simulink model "sim_2023_A2_inv_pend_OPT"  (R2022b)
settings: Solver=ode45  StartTime=0.0  StopTime=Tf  RelTol=1e-3
StartFcn:
  | sim_inv_pend
values from neighbouring files (symbols this model uses):
  A = sys_dt.A    [main_inv_pend.m]
  AN = [INm ... (first row only)    [gen_mpc_matrices.m]
  B = sys_dt.B    [main_inv_pend.m]
  C = sys_dt.C    [main_inv_pend.m]
  CL = 1    [main_inv_pend.m]
  controller = 1    [main_inv_pend.m]
  F = Phi'*QN*Lambda    [gen_mpc_matrices.m]
  Kf = Kf_t'    [main_inv_pend.m]
  Lambda = zeros(N*n,n)    [gen_mpc_matrices.m]
  N = 1    [gen_mpc_matrices.m]    (also in main_inv_pend.m = 16)
  noise = 1    [main_inv_pend.m]
  obs = 1    [main_inv_pend.m]
  saturate = 0    [main_inv_pend.m]
  th_o = 0    [main_inv_pend.m]
  Ts = 1/20    (= 0.05)    [main_inv_pend.m]
  Umax = [Umax;umax]    [gen_mpc_matrices.m]
  Umin = [Umin;umin]    [gen_mpc_matrices.m]
  W = 1*sqrt(M/5)    [animated_inv_pend_uw_clkw.m]    (also in gen_mpc_matrices.m = (W+W')/2)
  w_o = 0    [main_inv_pend.m]
  x_o = -1    [main_inv_pend.m]
  Xmax = [Xmax;xmax]    [gen_mpc_matrices.m]
  Xmin = [Xmin;xmin]    [gen_mpc_matrices.m]
  xo_hat = [0 0 0 0]'    [main_inv_pend.m]
  xsp_o = 0    [main_inv_pend.m]
undefined symbols (not defined in the file or in its folder): b, g, K, l, Mc, mp
settings Model: Creator=ricardoaguilera  LastModifiedBy=lucien
settings SolverCC: AlgebraicLoopSolver=TrustRegion
settings DataIOCC: ReturnWorkspaceOutputs=off
settings OptimizationCC: LifeSpan=inf
settings DebuggingCC: AlgebraicLoopMsg=none  UnconnectedInputMsg=warning  UnconnectedOutputMsg=warning  UnconnectedLineMsg=warning  SFMachineParentedDataDiag=warning  ArithmeticOperatorsInVariantConditions=warning
settings ModelReferenceCC: EnableRefExpFcnMdlSchedulingChecks=on
settings SFSimCC: CustomCodeUndefinedFunction=UseInterfaceOnly
settings RTWCC: DLArmComputeVersion=19.05
settings CodeAppCC: StateflowObjectComments=on

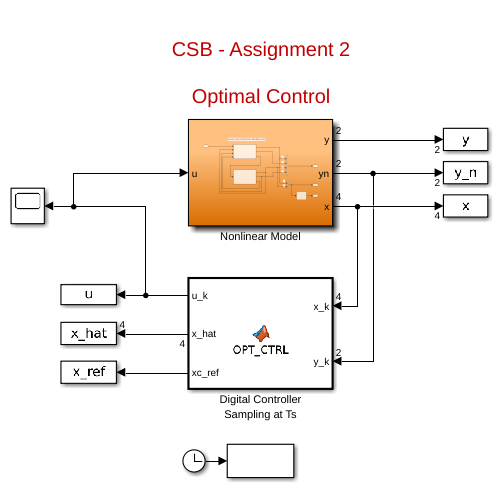
[thumbnail: Simulink's stored preview of the top-level diagram]
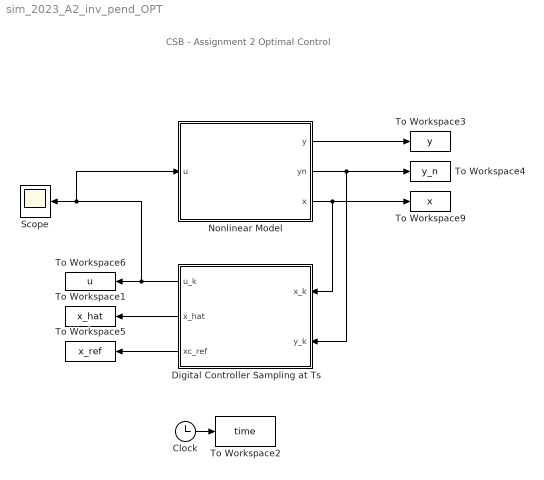
== system sim_2023_A2_inv_pend_OPT ==
  note: CSB - Assignment 2
      |
      | Optimal Control
  Clock : Clock
  Digital Controller Sampling at Ts : MATLAB Function  TreatAsAtomicUnit=on  SystemSampleTime=Ts
  Nonlinear Model : Subsystem
  Scope : Scope
  To Workspace1 : ToWorkspace  VariableName=x_hat  SampleTime=Ts/100
  To Workspace2 : ToWorkspace  VariableName=time  SampleTime=Ts/100
  To Workspace3 : ToWorkspace  VariableName=y  SampleTime=Ts/100
  To Workspace4 : ToWorkspace  VariableName=y_n  SampleTime=Ts/100
  To Workspace5 : ToWorkspace  VariableName=x_ref  SampleTime=Ts/100
  To Workspace6 : ToWorkspace  VariableName=u  SampleTime=Ts/100
  To Workspace9 : ToWorkspace  VariableName=x  SampleTime=Ts/100
  wires:
  Clock/1 -> To Workspace2/1
  Digital Controller Sampling at Ts/2(x_hat) -> To Workspace1/1
  Nonlinear Model/2(yn) -> Digital Controller Sampling at Ts/2(y_k), To Workspace4/1
  Nonlinear Model/3(x) -> Digital Controller Sampling at Ts/1(x_k), To Workspace9/1
  Nonlinear Model/1(y) -> To Workspace3/1
  Digital Controller Sampling at Ts/3(xc_ref) -> To Workspace5/1
  Digital Controller Sampling at Ts/1(u_k) -> To Workspace6/1, Nonlinear Model/1(u), Scope/1

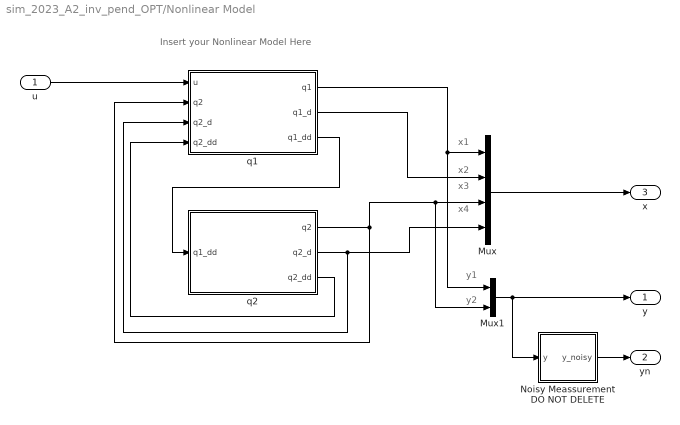
== system sim_2023_A2_inv_pend_OPT/Nonlinear Model ==
  note: x1
  note: Insert your Nonlinear Model Here
  note: x2
  note: x3
  note: x4
  note: y1
  note: y2
  u : Inport
  Mux : Mux
  Mux1 : Mux  Inputs=2
  Noisy Meassurement DO NOT DELETE : Subsystem
  q1 : Subsystem
  q2 : Subsystem
  y : Outport  VectorParamsAs1DForOutWhenUnconnected=off
  yn : Outport  Port=2  VectorParamsAs1DForOutWhenUnconnected=off
  x : Outport  Port=3  VectorParamsAs1DForOutWhenUnconnected=off
  wires:
  q2/3(q2_dd) -> q1/4(q2_dd)
  q2/2(q2_d) -> q1/3(q2_d), Mux/4
  q2/1(q2) -> q1/2(q2), Mux1/2, Mux/3
  q1/2(q1_d) -> Mux/2
  q1/1(q1) -> Mux1/1, Mux/1
  Mux/1 -> x/1
  Mux1/1 -> Noisy Meassurement DO NOT DELETE/1(y), y/1
  u/1 -> q1/1(u)
  Noisy Meassurement DO NOT DELETE/1(y_noisy) -> yn/1
  q1/3(q1_dd) -> q2/1(q1_dd)

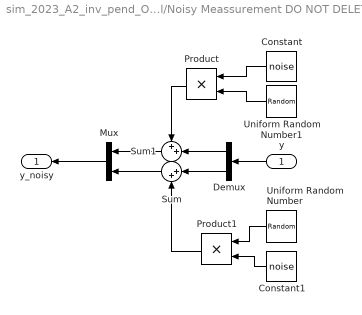
== system sim_2023_A2_inv_pend_OPT/Nonlinear Model/Noisy Meassurement DO NOT DELETE ==
  y : Inport
  Constant : Constant  Value=noise
  Constant1 : Constant  Value=noise
  Demux : Demux  Outputs=2
  Mux : Mux  Inputs=2
  Product : Product
  Product1 : Product
  Sum : Sum  Inputs=|++
  Sum1 : Sum  Inputs=++|
  Uniform Random Number : UniformRandomNumber  Minimum=-0.002  Maximum=0.002  SampleTime=0.5*Ts
  Uniform Random Number1 : UniformRandomNumber  Minimum=-0.3  Maximum=0.3  SampleTime=0.5*Ts
  y_noisy : Outport  VectorParamsAs1DForOutWhenUnconnected=off
  wires:
  Mux/1 -> y_noisy/1
  y/1 -> Demux/1
  Demux/2 -> Sum/1
  Sum/1 -> Mux/2
  Sum1/1 -> Mux/1
  Demux/1 -> Sum1/2
  Constant/1 -> Product/1
  Uniform Random Number1/1 -> Product/2
  Product/1 -> Sum1/1
  Product1/1 -> Sum/2
  Uniform Random Number/1 -> Product1/1
  Constant1/1 -> Product1/2

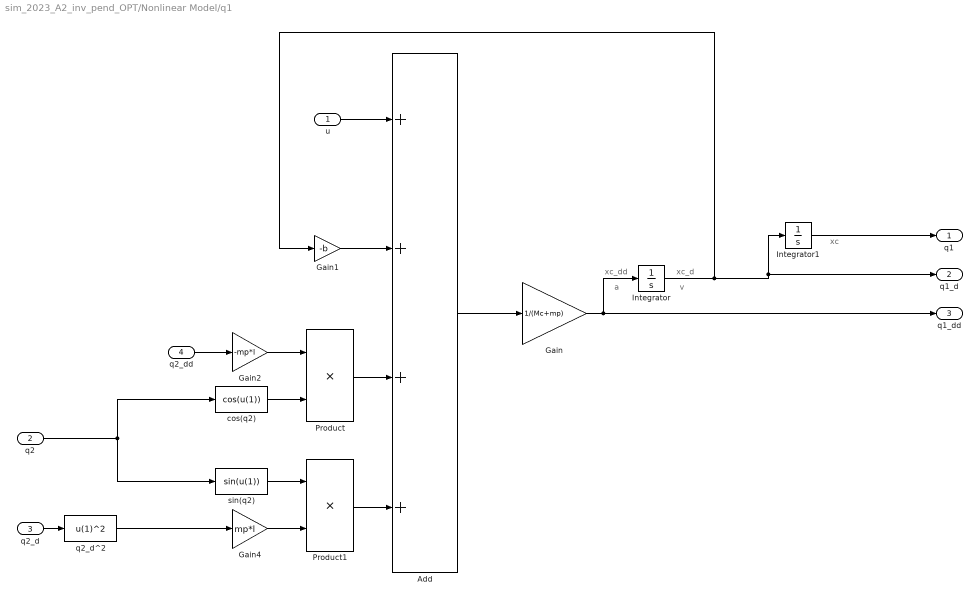
== system sim_2023_A2_inv_pend_OPT/Nonlinear Model/q1 ==
  note: a
  note: xc_dd
  note: v
  note: xc_d
  note: xc
  u : Inport
  q2 : Inport  Port=2
  q2_d : Inport  Port=3
  q2_dd : Inport  Port=4
  Add : Sum  Inputs=++++
  Gain : Gain  Gain=1/(Mc+mp)
  Gain1 : Gain  Gain=-b
  Gain2 : Gain  Gain=-mp*l
  Gain4 : Gain  Gain=mp*l
  Integrator : Integrator  InitialCondition=xsp_o
  Integrator1 : Integrator  InitialCondition=x_o
  Product : Product
  Product1 : Product
  cos(q2) : Fcn  Expr=cos(u(1))
  q2_d^2 : Fcn  Expr=u(1)^2
  sin(q2) : Fcn  Expr=sin(u(1))
  q1 : Outport  VectorParamsAs1DForOutWhenUnconnected=off
  q1_d : Outport  Port=2  VectorParamsAs1DForOutWhenUnconnected=off
  q1_dd : Outport  Port=3  VectorParamsAs1DForOutWhenUnconnected=off
  wires:
  Gain/1 -> Integrator/1, q1_dd/1
  Integrator1/1 -> q1/1
  Integrator/1 -> Gain1/1, q1_d/1, Integrator1/1
  Add/1 -> Gain/1
  u/1 -> Add/1
  Gain1/1 -> Add/2
  Product/1 -> Add/3
  Gain2/1 -> Product/1
  cos(q2)/1 -> Product/2
  Product1/1 -> Add/4
  sin(q2)/1 -> Product1/1
  Gain4/1 -> Product1/2
  q2_d/1 -> q2_d^2/1
  q2_d^2/1 -> Gain4/1
  q2/1 -> sin(q2)/1, cos(q2)/1
  q2_dd/1 -> Gain2/1

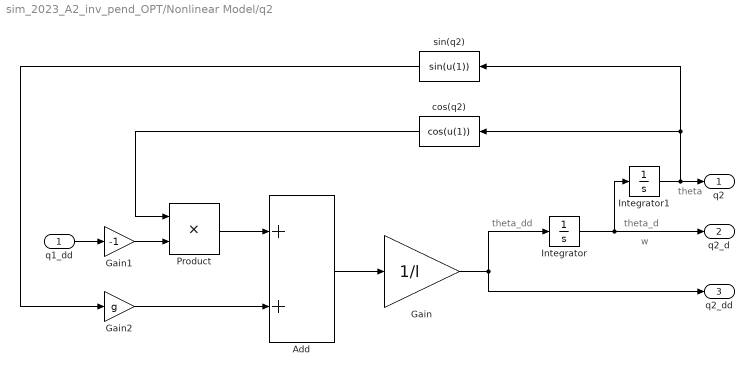
== system sim_2023_A2_inv_pend_OPT/Nonlinear Model/q2 ==
  note: theta_dd
  note: w
  note: theta_d
  note: theta
  q1_dd : Inport
  Add : Sum
  Gain : Gain  Gain=1/l
  Gain1 : Gain  Gain=-1
  Gain2 : Gain  Gain=g
  Integrator : Integrator  InitialCondition=w_o
  Integrator1 : Integrator  InitialCondition=th_o
  Product : Product
  cos(q2) : Fcn  Expr=cos(u(1))
  sin(q2) : Fcn  Expr=sin(u(1))
  q2 : Outport  VectorParamsAs1DForOutWhenUnconnected=off
  q2_d : Outport  Port=2  VectorParamsAs1DForOutWhenUnconnected=off
  q2_dd : Outport  Port=3  VectorParamsAs1DForOutWhenUnconnected=off
  wires:
  Gain/1 -> q2_dd/1, Integrator/1
  Integrator1/1 -> sin(q2)/1, cos(q2)/1, q2/1
  Integrator/1 -> q2_d/1, Integrator1/1
  q1_dd/1 -> Gain1/1
  Add/1 -> Gain/1
  Gain1/1 -> Product/2
  cos(q2)/1 -> Product/1
  sin(q2)/1 -> Gain2/1
  Gain2/1 -> Add/2
  Product/1 -> Add/1

== matlab function sim_2023_A2_inv_pend_OPT/Digital Controller Sampling at Ts ==
  data: x_k input; y_k input; u_k output; xo_hat parameter; obs parameter; CL parameter; x_hat output; controller parameter; Kf parameter; K parameter; A parameter; B parameter; C parameter; W parameter; F parameter; xc_ref output; N parameter; Lambda parameter; Umin parameter; Umax parameter; Xmax parameter; Xmin parameter; AN parameter; saturate parameter
function [u_k,x_hat, xc_ref]= OPT_CTRL(x_k,y_k,xo_hat,obs, CL, controller, Kf, K, A, B, C, W, F, N, Lambda, Umin, Umax, Xmax, Xmin, AN, saturate)
%% Instructions CSB A2
%
% 1) This block will run every Ts
%
% 2) It is possible to read variables from workspase.
%    For example, to read matrix A, add it to fcn(x_k,A).
%    Then go to Edit Data (next to Build MOdel)and chage 
%    its "Scope" in the left-hand side from Output to Parameter.
%
% 3) To avoid simulation erros, initialise anyblock output variable with
%    the rigth dimension.
%
% 4) Use persistent to declare variables that needs to be memorised.
%
%% Required Quadprog settings: DO NOT DELETE
coder.extrinsic('quadprog');        %Required to be called from Simulink
opts=  optimset('display','off');   %not displaying quadprog messages in the workspace
exitflag=0;
persistent one_message
if isempty(one_message)
    one_message=0;
end

%% System dimensions
n=length(A);
m=size(B)*[0 1]';

%% Initializing block outputs signals and Optimal vector
u_k=0;              %Do not delete
x_hat=zeros(4,1);   %Do not delete
Uopt=zeros(N,m);    %Do not delete


%% Use persistent for variables that requiered to be momorised
persistent x_hat_k
if isempty(x_hat_k)
    x_hat_k = xo_hat;   % Kalman filter initial condition (change in main)
end
persistent count        % Counter for step reference
    if isempty(count)
        count = 0;
    end
x_hat=x_hat_k;  %Send out the kalman filter estimate


%% Creating a Step-Changing Reference for the cart position
% DO NOT CHANGE THIS REFERENCE
y_ref=zeros(2,1);
xc_ref= 1;  %Reference for cart position
if count>300
   xc_ref=5; %Reference for cart position
end
count=count+1;
if count==600
    count=0;
end
y_ref(1)=xc_ref;    %Reference for cart position
y_ref(2)=0;         %Reference for pendulum angle

%% Optimal Control
if (CL==1)
    x_ref=[y_ref(1) 0 y_ref(2) 0]';
    if (obs==1)
        x=x_hat_k;  %Optimal Controller will use the system state estimates
    else
        x=x_k;      %Optimal Controller will use the actual system states
    end
    
    
    switch controller
    case 1  %LQR
        %% Implement your LQR here
        u_ref = 0;
        u_k= -K*(x-x_ref) + u_ref;
        if (saturate > 0)
            if (u_k > 15.0)
                u_k = 15;
            elseif (u_k < -15)
                u_k = -15;
            end
        end
    case 2  %MPC
        
        %% CHANGE the matrices below accordingly 
        H=2*W;              %Compute Hessian for your MPC design
        xe=(x-x_ref);         %Initial tracking error
        f= 2 * F *xe;   %Compute f vector for your MPC design
        
        bN=[ Umax;
           -Umin;
            Xmax;
           -Xmin];
       %%
       % After properly adding the required matrices, quadprog will find
       % the optimal input vector as per below.
                         %X = quadprog(H,f,A, b, Aeq,beq,LB,UB,X0,OPTIONS) from help quadprog
        [Uopt,fval,exitflag]= quadprog(H,f,AN,bN,[] ,[] ,[],[],[],opts); %DO NOT CHANGE THIS
    
        %exitflag is used to vefied whether a feasible solution has been found
        if (exitflag>0)
            %Feasible solution has been found then, apply first actuation
            u_k=Uopt(1);    
        else
            %Feasible solution has NOT been found then, apply uncosntrained
            %optimal solution
            if (one_message==0)
                disp(' ');
                disp('No feasible solution has been found:')
                disp('Try again increasing the predictoin horizon N')
                disp(' ')
                one_message=1;
            end
            Uopt=-inv(W)*F*xe; %Unconstrained solution
            u_k=Uopt(1);
        end
    end
    %% Implement your Kalman Filter (KF) here
    % KF is common for bor LQR and MPC
    y_hat_k = C*x_hat_k;
    x_hat_k=A*x_hat_k+B*u_k+Kf*(y_k-y_hat_k);
else
    u_k=0;  %for open-loop
end
